simulink model "jointInvDyn"  (R2021b)
settings: Solver=VariableStepAuto  StartTime=0.0  StopTime=3  RelTol=1e-3
undefined symbols (not defined in the file): Kd, Kp
libraries: robotcorelib x1, simulink x1
settings Model: Creator=fabio  LastModifiedBy=buse

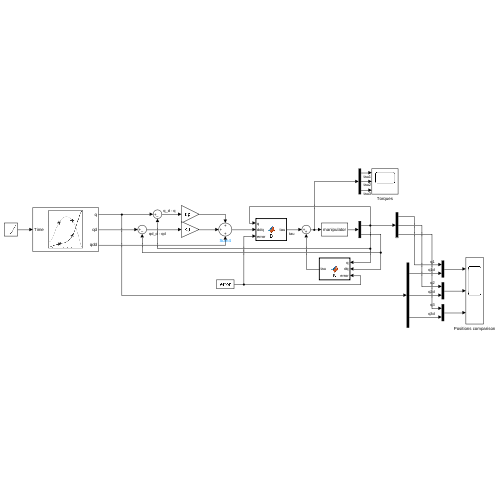
[thumbnail: Simulink's stored preview of the top-level diagram]
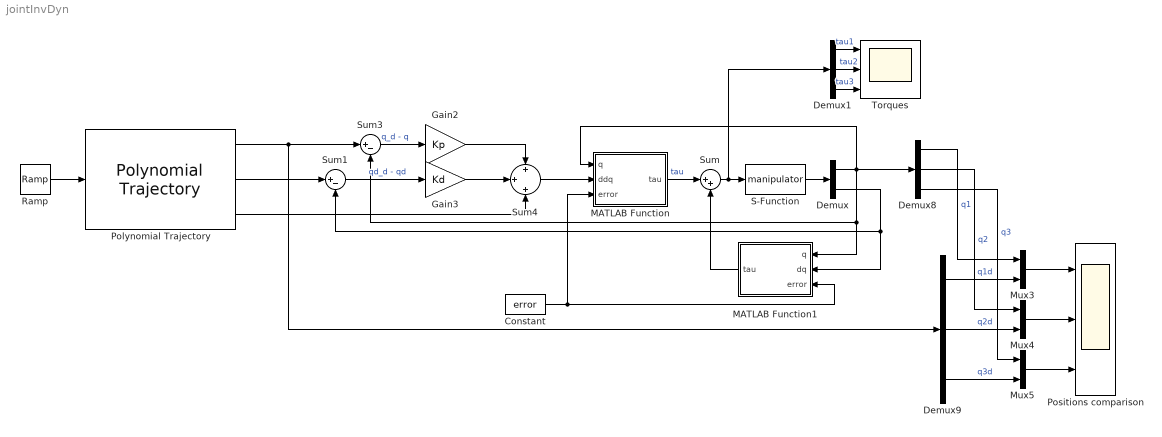
== system jointInvDyn ==
  Constant : Constant  Value=error
  Demux : Demux  Outputs=2
  Demux1 : Demux  Outputs=3
  Demux8 : Demux  Outputs=3
  Demux9 : Demux  Outputs=3
  Gain2 : Gain  Gain=Kp
  Gain3 : Gain  Gain=Kd
  MATLAB Function : MATLAB Function  TreatAsAtomicUnit=on
  MATLAB Function1 : MATLAB Function  TreatAsAtomicUnit=on
  Mux3 : Mux  Inputs=2
  Mux4 : Mux  Inputs=2
  Mux5 : Mux  Inputs=2
  Polynomial Trajectory : robotcorelib/Polynomial Trajectory  WaypointSource=Internal  Waypoints=wpts  TimePoints=time  TimeInterval=[ 1, 4 ]  Method=Quintic Polynomial  ParameterSource=Internal  VelocityBoundaryCondition=velBound  AccelerationBoundaryCondition=accBound  SimulateUsing=Interpreted execution
  Positions comparison : Scope  NumInputPorts=3
  Ramp : simulink/Sources/Ramp  slope=1  start=0  InitialOutput=0
  S-Function : S-Function  FunctionName=manipulator  Parameters=robot  SFunctionDeploymentMode=off  EnableBusSupport=off
  Sum : Sum  Inputs=|++
  Sum1 : Sum  Inputs=|+-
  Sum3 : Sum  Inputs=|+-
  Sum4 : Sum  Inputs=+|+|+
  Torques : Scope  NumInputPorts=3
  wires:
  Demux9/2 -> Mux4/2  "q2d"
  Mux4/1 -> Positions comparison/2
  Mux3/1 -> Positions comparison/1
  Demux9/3 -> Mux5/2  "q3d"
  Sum3/1 -> Gain2/1  "q_d - q"
  Demux9/1 -> Mux3/2  "q1d"
  Demux8/2 -> Mux4/1  "q2"
  Demux8/3 -> Mux5/1  "q3"
  S-Function/1 -> Demux/1
  Demux8/1 -> Mux3/1  "q1"
  Mux5/1 -> Positions comparison/3
  Demux/1 -> MATLAB Function/1(q), Demux8/1, MATLAB Function1/1(q), Sum3/2
  Gain2/1 -> Sum4/1
  Gain3/1 -> Sum4/2
  Sum1/1 -> Gain3/1  "qd_d - qd"
  Demux/2 -> MATLAB Function1/2(dq), Sum1/2
  Sum4/1 -> MATLAB Function/2(ddq)
  Sum/1 -> Demux1/1, S-Function/1
  MATLAB Function/1(tau) -> Sum/1  "tau"
  MATLAB Function1/1(tau) -> Sum/2
  Ramp/1 -> Polynomial Trajectory/1
  Polynomial Trajectory/1 -> Demux9/1, Sum3/1
  Polynomial Trajectory/2 -> Sum1/1
  Polynomial Trajectory/3 -> Sum4/3
  Demux1/1 -> Torques/1  "tau1"
  Demux1/2 -> Torques/2  "tau2"
  Demux1/3 -> Torques/3  "tau3"
  Constant/1 -> MATLAB Function1/3(error), MATLAB Function/3(error)

== matlab function jointInvDyn/MATLAB Function1 ==
  data: q input size=3; tau output; dq input size=3; error input
function tau = N(q, dq, error)
    q1 = q(1); q2 = q(2); q3 = q(3);
    dq1 = dq(1); dq2 = dq(2); dq3 = dq(3);
    if error == 0
        tau = [dq3*(0.03923*cos(q3)*dq3^2 - 0.5*dq1*(0.0474*sin(2.0*q3) + 0.05885*sin(q3) + 0.1962*q2*sin(q3))*dq3) - 1.0*dq1*(0.5*dq3^2*(0.0474*sin(2.0*q3) + 0.05885*sin(q3) + 0.1962*q2*sin(q3)) - 0.5*dq2^2*(3.098*q2 + 0.1962*cos(q3) + 0.7099)) + 0.5*dq1*dq2^2*(3.098*q2 + 0.1962*cos(q3) + 0.7099);
            0.5*dq1^2*dq2*(3.098*q2 + 0.1962*cos(q3) + 0.7099);
            0.9621*cos(q3) + dq1*(0.03923*cos(q3)*dq3^2 - 0.5*dq1*(0.0474*sin(2.0*q3) + 0.05885*sin(q3) + 0.1962*q2*sin(q3))*dq3)];
    else
        tau = [dq3*(0.0336*cos(q3)*dq3^2 - 0.5*dq1*(0.0406*sin(2.0*q3) + 0.0504*sin(q3) + 0.168*q2*sin(q3))*dq3) - 1.0*dq1*(0.5*dq3^2*(0.0406*sin(2.0*q3) + 0.0504*sin(q3) + 0.168*q2*sin(q3)) - 0.5*dq2^2*(2.4*q2 + 0.168*cos(q3) + 0.57)) + 0.5*dq1*dq2^2*(2.4*q2 + 0.168*cos(q3) + 0.57);
        0.5*dq1^2*dq2*(2.4*q2 + 0.168*cos(q3) + 0.57);
        0.824*cos(q3) + dq1*(0.0336*cos(q3)*dq3^2 - 0.5*dq1*(0.0406*sin(2.0*q3) + 0.0504*sin(q3) + 0.168*q2*sin(q3))*dq3)];
    end
end

== matlab function jointInvDyn/MATLAB Function ==
  data: q input size=3; tau output; ddq input size=3; error input
function tau = B(q, ddq, error)
    q1 = q(1); q2 = q(2); q3 = q(3);
    if error == 0
        B = [0.7099*q2 + 0.05885*cos(q3) + 0.0474*cos(q3)^2 + 0.1962*q2*cos(q3) + 1.549*q2^2 + 0.496,          -0.6196,  0.03923*sin(q3);
            -0.6196,            1.549, -0.09808*sin(q3);
     0.03923*sin(q3), -0.09808*sin(q3),          0.04757];
    else
        B = [0.57*q2 + 0.0504*cos(q3) + 0.0406*cos(q3)^2 + 0.168*q2*cos(q3) + 1.2*q2^2 + 0.3857,          -0.48, 0.0336*sin(q3);
            -0.48,            1.2, -0.084*sin(q3);
            0.0336*sin(q3), -0.084*sin(q3),        0.04074];
    end
    tau = B*ddq;
